simulink model "HIL_2"  (R2024a)
settings: Solver=ode3  StartTime=0.0  StopTime=inf  FixedStep=0.01  RelTol=1e-3  EnableMultiTasking=on
undefined symbols (not defined in the file or in its folder): k
libraries: arduinolib x3, simulink x2
settings Model: FPTRunName=Active  SimulationMode=external  ExtModeTrigDuration=2  Creator=refai  LastModifiedBy=refai
settings SolverCC: AlgebraicLoopSolver=TrustRegion  AutoInsertRateTranBlk=on
settings DataIOCC: LimitDataPoints=on  SaveFormat=Array
settings OptimizationCC: ReuseModelBlockBuffer=off  ExpressionDepthLimit=2147483647  LifeSpan=Inf  MaxStackSize=64
settings DebuggingCC: UnderspecifiedInitializationDetection=Classic  MergeDetectMultiDrivingBlocksExec=none  FcnCallInpInsideContextMsg=warning  UnconnectedInputMsg=warning  UnconnectedOutputMsg=warning  UnconnectedLineMsg=warning  AllowSymbolicDim=off  StateNameClashWarn=warning  SFUnexpectedBacktrackingDiag=warning  SFNoUnconditionalDefaultTransitionDiag=warning  SFExecutionAtInitializationDiag=none  ArithmeticOperatorsInVariantConditions=warning
settings HardwareCC: ProdBitPerInt=16  ProdBitPerPointer=16  ProdBitPerSizeT=16  ProdBitPerPtrDiffT=16  ProdLargestAtomicFloat=None  ProdWordSize=8  ProdHWDeviceType=Atmel->AVR
settings ModelReferenceCC: EnableRefExpFcnMdlSchedulingChecks=on  PropagateSignalLabelsOutOfModel=off
settings SFSimCC: SimUseLocalCustomCode=off  CustomCodeUndefinedFunction=UseInterfaceOnly
settings RTWCC: Description=Embedded Coder  SystemTargetFile=ert.tlc  HardwareBoard=Arduino Uno  TemplateMakefile=ert_default_tmf  GenerateReport=on  RTWVerbose=off  RTWUseLocalCustomCode=off  Toolchain=Arduino AVR  BuildConfiguration=Faster Runs  LaunchReport=on  GPUComputeCapability=3.5
settings CodeAppCC: ForceParamTrailComments=on  OperatorAnnotations=on  StateflowObjectComments=on  MATLABSourceComments=on
settings ERTTargetCC: MultiwordLength=2048  ERTCustomFileBanners=off  SupportContinuousTime=on  SupportNonInlinedSFcns=on  RemoveResetFunc=off  SupportVariableSizeSignals=on  ModelStepFunctionPrototypeControlCompliant=off  ExtMode=on  ExtModeTransport=3  ExtModeStaticAlloc=on  ExtModeAutomaticAllocSize=off  ExtModeStaticAllocSize=250  ExtModeMexFile=ext_xcp  ExtModeMexArgs=0 8 115200  ExtModeIntrfLevel=Level2 - Open
settings ConfigComp: CovMetricSettings=dw  CovSaveCumulativeToWorkspaceVar=on  CovSaveSingleToWorkspaceVar=on  CovExternalEMLEnable=off  CovSFcnEnable=off

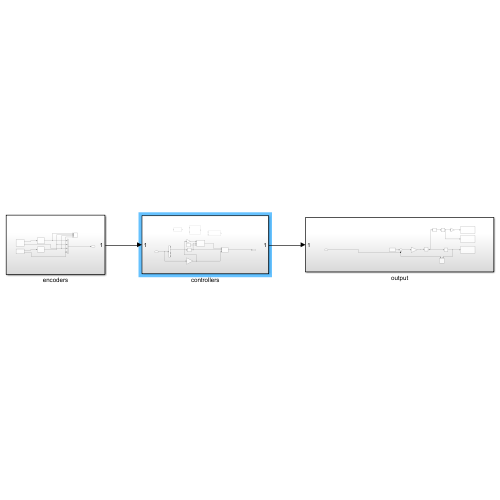
[thumbnail: Simulink's stored preview of the top-level diagram]
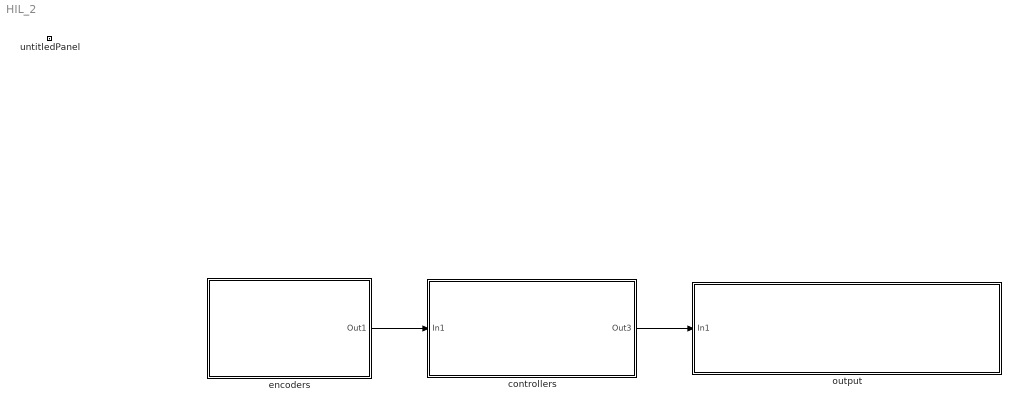
== system HIL_2 ==
  controllers : Subsystem
  encoders : Subsystem
  output : Subsystem
  untitledPanel : Subsystem  Tag=HiddenForWebPanel  IsWebBlockPanel=on
  wires:
  encoders/1(Out1) -> controllers/1(In1)
  controllers/1(Out3) -> output/1(In1)

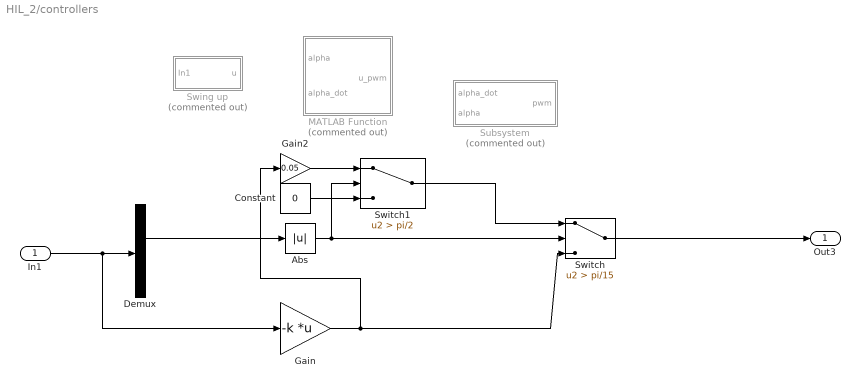
== system HIL_2/controllers ==
  In1 : Inport
  Abs : Abs  SaturateOnIntegerOverflow=off
  Constant : Constant  Value=0
  Demux : Demux
  Gain : Gain  Gain=-k  Multiplication=Matrix(K*u) (u vector)  ParamDataTypeStr=single  OutDataTypeStr=single
  Gain2 : Gain  Gain=0.05
  MATLAB Function : MATLAB Function  Commented=on  TreatAsAtomicUnit=on
  Subsystem : Subsystem  Commented=on
  Swing up : Subsystem  Commented=on
  Switch : Switch  Criteria=u2 > Threshold  Threshold=pi/15  SaturateOnIntegerOverflow=off  InputSameDT=off
  Switch1 : Switch  Criteria=u2 > Threshold  Threshold=pi/2  SaturateOnIntegerOverflow=off  InputSameDT=off
  Out3 : Outport
  wires:
  Gain/1 -> Gain2/1, Switch/3
  Abs/1 -> Switch1/2, Switch/2
  Demux/2 -> Abs/1
  In1/1 -> Demux/1, Gain/1
  Switch/1 -> Out3/1
  Gain2/1 -> Switch1/1
  Constant/1 -> Switch1/3
  Switch1/1 -> Switch/1

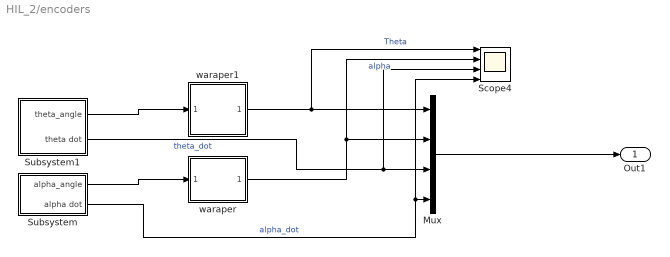
== system HIL_2/encoders ==
  Mux : Mux
  Scope4 : Scope  NumInputPorts=4
  Subsystem : Subsystem
  Subsystem1 : Subsystem
  waraper : Subsystem
  waraper1 : Subsystem
  Out1 : Outport
  wires:
  Subsystem1/2(theta dot) -> Scope4/3, Mux/3  "theta_dot"
  Subsystem/2(alpha dot) -> Mux/4, Scope4/4  "alpha_dot"
  waraper/1(Output) -> Mux/2, Scope4/2  "alpha"
  Subsystem1/1(theta_angle) -> waraper1/1(Input)
  waraper1/1(Output) -> Scope4/1, Mux/1  "Theta"
  Subsystem/1(alpha_angle) -> waraper/1(Input)
  Mux/1 -> Out1/1

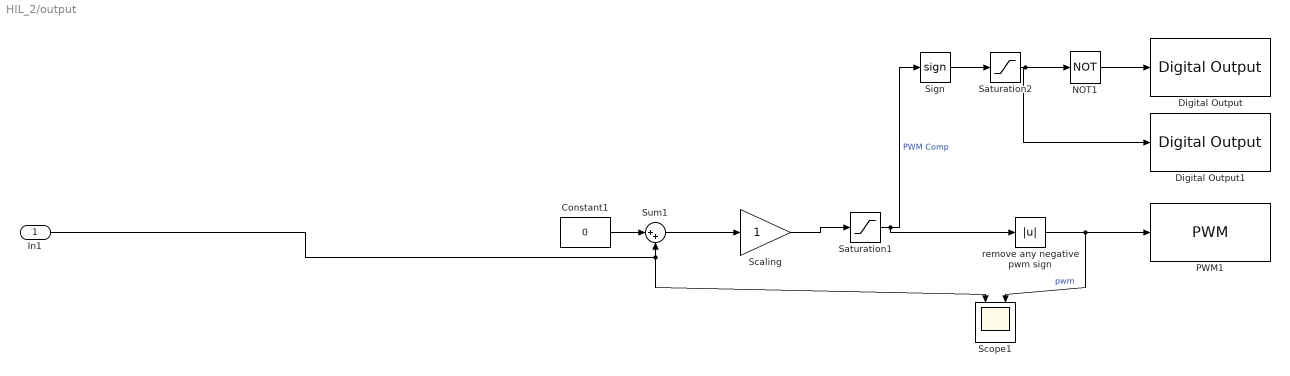
== system HIL_2/output ==
  In1 : Inport
  Constant1 : Constant  Value=0
  Digital Output : arduinolib/Digital Output  pinNumber=7  Direction=output  blockPlatform=arduino
  Digital Output1 : arduinolib/Digital Output  pinNumber=8  Direction=output  blockPlatform=arduino
  NOT1 : Logic  Operator=NOT  IconShape=distinctive  AllPortsSameDT=off  OutDataTypeStr=boolean
  PWM1 : arduinolib/PWM  pinNumber=9  frequencyType=Default  desiredFrequency=490.2  achievableFrequency=490.2
  Saturation1 : Saturate  UpperLimit=255  LowerLimit=-255
  Saturation2 : Saturate  UpperLimit=1  LowerLimit=0
  Scaling : Gain
  Scope1 : Scope  NumInputPorts=2
  Sign : Signum
  Sum1 : Sum  Inputs=|++
  remove any negative pwm sign : Abs  SaturateOnIntegerOverflow=off
  wires:
  Saturation2/1 -> Digital Output1/1, NOT1/1
  Scaling/1 -> Saturation1/1
  NOT1/1 -> Digital Output/1
  Sum1/1 -> Scaling/1
  Sign/1 -> Saturation2/1
  Saturation1/1 -> remove any negative pwm sign/1, Sign/1  "PWM Comp"
  In1/1 -> Scope1/1, Sum1/2
  remove any negative pwm sign/1 -> PWM1/1, Scope1/2  "pwm"
  Constant1/1 -> Sum1/1

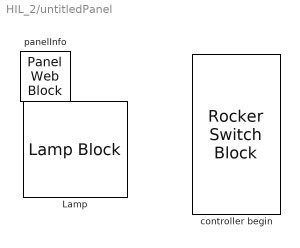
== system HIL_2/untitledPanel ==
  Lamp : LampBlock  Tag=HiddenForWebPanel  PanelInfo="{\"height\":158,\"left\":30,\"panelId\":\"panelId-8c924346-006a-4594-a17e-8cf792d8abfa\",\"top\":107,\"type\":\"panelChild\",\"version\":\"2019b\",\"width\":171,\"zIndex\":1500002}"  LabelPosition=Hide
  controller begin : RockerSwitchBlock  Tag=HiddenForWebPanel  PanelInfo="{\"height\":263,\"left\":308,\"panelId\":\"panelId-8c924346-006a-4594-a17e-8cf792d8abfa\",\"top\":30,\"type\":\"panelChild\",\"version\":\"2019b\",\"width\":145,\"zIndex\":1500004}"
      settings: Values={{'Off', 'On'}, [0 1]}
  panelInfo : PanelWebBlock  Tag=HiddenForWebPanel  PanelInfo="{\"compacted\":false,\"height\":329,\"isActiveTab\":true,\"left\":505,\"name\":\"Panel\",\"panelId\":\"panelId-8c924346-006a-4594-a17e-8cf792d8abfa\",\"popoutData\":{\"height\":0,\"left\":0,\"maximized\":false,\"top\":0,\"width\":0},\"popoutMode\":\"component\",\"tabIndex\":0,\"tabbedSetId\":\"tabbedSet4765928719\",\"top\":34,\"type\":\"panel\",\"version\":\"2019b\",\"visible\":true,\"width\":489,\"zIndex\":1500002}"  PanelSnapshot=<binary blob, 652 chars, not shown>

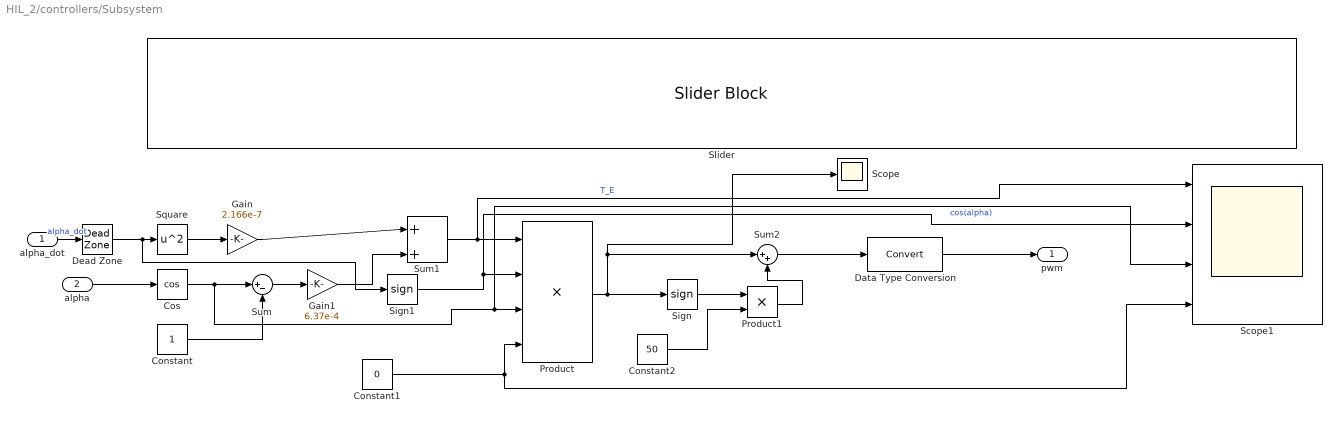
== system HIL_2/controllers/Subsystem ==
  alpha_dot : Inport
  alpha : Inport  Port=2
  Constant : Constant
  Constant1 : Constant  Value=0
  Constant2 : Constant  Value=50
  Cos : Trigonometry  Operator=cos
  Data Type Conversion : DataTypeConversion  SaturateOnIntegerOverflow=off  RndMeth=Floor
  Dead Zone : DeadZone
  Gain : Gain  Gain=2.166e-7
  Gain1 : Gain  Gain=6.37e-4
  Product : Product  Inputs=4
  Product1 : Product
  Scope : Scope
  Scope1 : Scope  NumInputPorts=4
  Sign : Signum
  Sign1 : Signum
  Slider : SliderBlock  ScaleMin=-100000  ScaleMax=100000
  Square : Math  Operator=square
  Sum : Sum  Inputs=|+-
  Sum1 : Sum  Inputs=|++
  Sum2 : Sum  Inputs=|++
  pwm : Outport  OutDataTypeStr=single
  wires:
  alpha_dot/1 -> Dead Zone/1  "alpha_dot"
  Square/1 -> Gain/1
  alpha/1 -> Cos/1
  Cos/1 -> Scope1/3, Product/3, Sum/1  "cos(alpha)"
  Constant/1 -> Sum/2
  Sum/1 -> Gain1/1
  Gain/1 -> Sum1/1
  Gain1/1 -> Sum1/2
  Sum1/1 -> Scope1/1, Product/1  "T_E"
  Constant1/1 -> Product/4, Scope1/4
  Product/1 -> Sign/1, Sum2/1, Scope/1
  Constant2/1 -> Product1/2
  Sign/1 -> Product1/1
  Product1/1 -> Sum2/2
  Sum2/1 -> Data Type Conversion/1
  Data Type Conversion/1 -> pwm/1
  Sign1/1 -> Scope1/2, Product/2
  Dead Zone/1 -> Sign1/1, Square/1

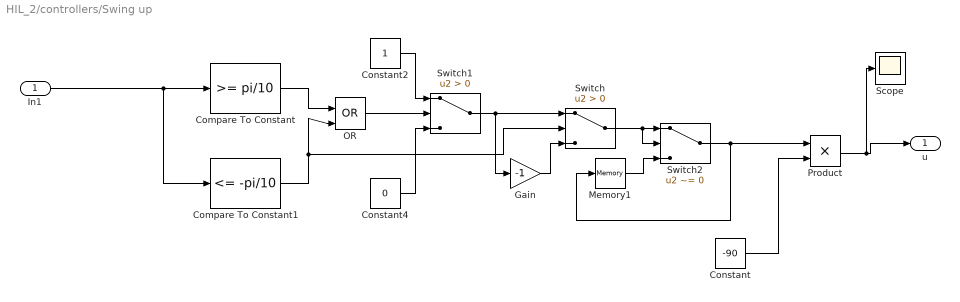
== system HIL_2/controllers/Swing up ==
  In1 : Inport
  Compare To Constant : simulink/Logic and Bit Operations/Compare To Constant  relop=>=  const=pi/10  OutDataTypeStr=boolean
  Compare To Constant1 : simulink/Logic and Bit Operations/Compare To Constant  relop=<=  const=-pi/10  OutDataTypeStr=boolean
  Constant : Constant  Value=-90
  Constant2 : Constant
  Constant4 : Constant  Value=0
  Gain : Gain  Gain=-1
  Memory1 : Memory  InitialCondition=1
  OR : Logic  Operator=OR  IconShape=distinctive  AllPortsSameDT=off  OutDataTypeStr=boolean
  Product : Product
  Scope : Scope
  Switch : Switch  Criteria=u2 > Threshold  SaturateOnIntegerOverflow=off  InputSameDT=off
  Switch1 : Switch  Criteria=u2 > Threshold  SaturateOnIntegerOverflow=off  InputSameDT=off
  Switch2 : Switch  Criteria=u2 ~= 0  SaturateOnIntegerOverflow=off  InputSameDT=off
  u : Outport
  wires:
  Switch1/1 -> Gain/1, Switch/1
  In1/1 -> Compare To Constant1/1, Compare To Constant/1
  Constant4/1 -> Switch1/3
  Constant2/1 -> Switch1/1
  Compare To Constant1/1 -> Switch/2, OR/2
  Compare To Constant/1 -> OR/1
  Gain/1 -> Switch/3
  OR/1 -> Switch1/2
  Constant/1 -> Product/2
  Switch/1 -> Switch2/2, Switch2/1
  Product/1 -> Scope/1, u/1
  Switch2/1 -> Product/1, Memory1/1
  Memory1/1 -> Switch2/3

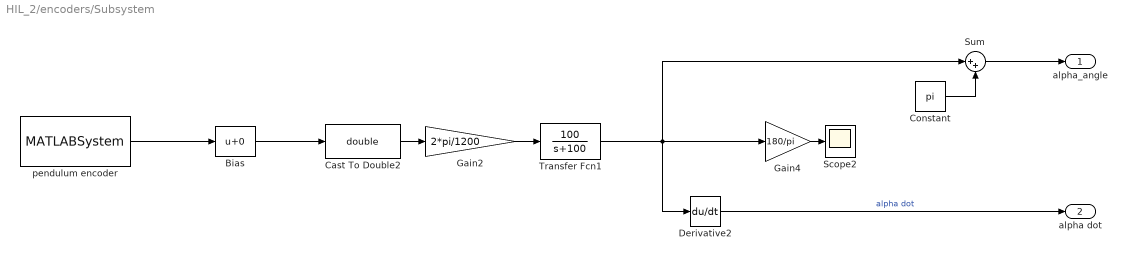
== system HIL_2/encoders/Subsystem ==
  Bias : Bias  SaturateOnIntegerOverflow=off
  Cast To Double2 : DataTypeConversion  OutDataTypeStr=double  SaturateOnIntegerOverflow=off  RndMeth=Floor
  Constant : Constant  Value=pi
  Derivative2 : Derivative
  Gain2 : Gain  Gain=2*pi/1200
  Gain4 : Gain  Gain=180/pi
  Scope2 : Scope
  Sum : Sum  Inputs=|++
  Transfer Fcn1 : TransferFcn  Numerator=[100]  Denominator=[1 100]
  pendulum encoder : MATLABSystem  System=Encoder_arduino  Encoder=0  PinA=3  PinB=5  SampleTime=0.01
      mask Type: Encoder_arduino
      mask Display:
      | disp('Encoder');
      | port_label('output',1,'y');
  alpha_angle : Outport
  alpha dot : Outport  Port=2
  wires:
  Transfer Fcn1/1 -> Sum/1, Gain4/1, Derivative2/1
  Gain2/1 -> Transfer Fcn1/1
  pendulum encoder/1 -> Bias/1
  Constant/1 -> Sum/2
  Gain4/1 -> Scope2/1
  Bias/1 -> Cast To Double2/1
  Cast To Double2/1 -> Gain2/1
  Sum/1 -> alpha_angle/1
  Derivative2/1 -> alpha dot/1  "alpha dot"

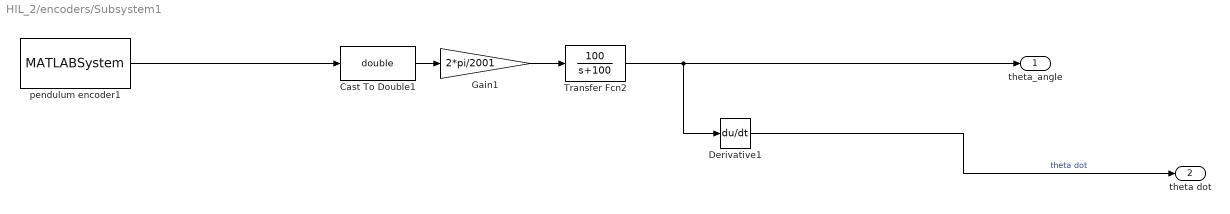
== system HIL_2/encoders/Subsystem1 ==
  Cast To Double1 : DataTypeConversion  OutDataTypeStr=double  SaturateOnIntegerOverflow=off  RndMeth=Floor
  Derivative1 : Derivative
  Gain1 : Gain  Gain=2*pi/2001
  Transfer Fcn2 : TransferFcn  Numerator=[100]  Denominator=[1 100]
  pendulum encoder1 : MATLABSystem  System=Encoder_arduino  Encoder=1  PinA=2  PinB=4  SampleTime=0.01
      mask Type: Encoder_arduino
      mask Display:
      | disp('Encoder');
      | port_label('output',1,'y');
  theta_angle : Outport
  theta dot : Outport  Port=2
  wires:
  Derivative1/1 -> theta dot/1  "theta dot"
  Transfer Fcn2/1 -> theta_angle/1, Derivative1/1
  pendulum encoder1/1 -> Cast To Double1/1
  Gain1/1 -> Transfer Fcn2/1
  Cast To Double1/1 -> Gain1/1

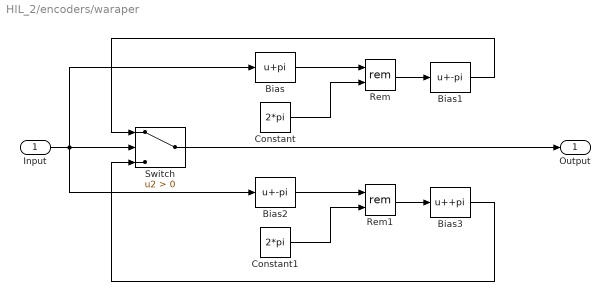
== system HIL_2/encoders/waraper ==
  Input : Inport
  Bias : Bias  Bias=pi  SaturateOnIntegerOverflow=off
  Bias1 : Bias  Bias=-pi  SaturateOnIntegerOverflow=off
  Bias2 : Bias  Bias=-pi  SaturateOnIntegerOverflow=off
  Bias3 : Bias  Bias=+pi  SaturateOnIntegerOverflow=off
  Constant : Constant  Value=2*pi
  Constant1 : Constant  Value=2*pi
  Rem : Math  Operator=rem
  Rem1 : Math  Operator=rem
  Switch : Switch  Criteria=u2 > Threshold  SaturateOnIntegerOverflow=off  InputSameDT=off
  Output : Outport
  wires:
  Constant/1 -> Rem/2
  Bias/1 -> Rem/1
  Input/1 -> Bias/1, Bias2/1, Switch/2
  Bias3/1 -> Switch/3
  Bias2/1 -> Rem1/1
  Rem1/1 -> Bias3/1
  Constant1/1 -> Rem1/2
  Switch/1 -> Output/1
  Rem/1 -> Bias1/1
  Bias1/1 -> Switch/1

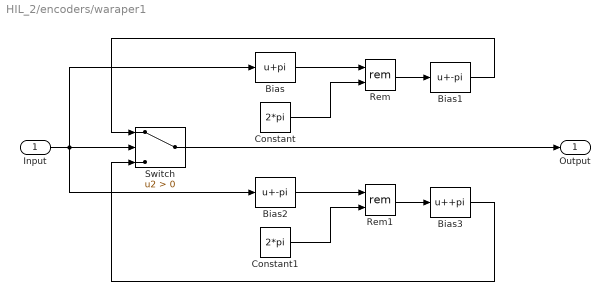
== system HIL_2/encoders/waraper1 ==
  Input : Inport
  Bias : Bias  Bias=pi  SaturateOnIntegerOverflow=off
  Bias1 : Bias  Bias=-pi  SaturateOnIntegerOverflow=off
  Bias2 : Bias  Bias=-pi  SaturateOnIntegerOverflow=off
  Bias3 : Bias  Bias=+pi  SaturateOnIntegerOverflow=off
  Constant : Constant  Value=2*pi
  Constant1 : Constant  Value=2*pi
  Rem : Math  Operator=rem
  Rem1 : Math  Operator=rem
  Switch : Switch  Criteria=u2 > Threshold  SaturateOnIntegerOverflow=off  InputSameDT=off
  Output : Outport
  wires:
  Constant/1 -> Rem/2
  Bias/1 -> Rem/1
  Input/1 -> Bias/1, Bias2/1, Switch/2
  Bias3/1 -> Switch/3
  Bias2/1 -> Rem1/1
  Rem1/1 -> Bias3/1
  Constant1/1 -> Rem1/2
  Switch/1 -> Output/1
  Rem/1 -> Bias1/1
  Bias1/1 -> Switch/1

== matlab function HIL_2/controllers/MATLAB Function ==
  data: alpha input; u_pwm output; alpha_dot input
function u_pwm = aggressive_swingup(alpha, alpha_dot)
    % --- INITIALIZATION ---
    % We use 'single' to ensure compatibility with Arduino hardware
    u_pwm = single(0);
    
    % --- CONFIGURATION ---
    % Power gain: 200-255 is aggressive for a 13g pendulum
    % If the motor 'brakes' instead of 'pushes', change this to -220
    ke = single(220); 
    
    % --- RANGE LOGIC (QUADRANT CONTROL) ---
    % Since alpha is wrapped between -pi and pi, the bottom half is 
    % split into two ranges
    
    % Range 1: Bottom-Right (90 to 180 degrees)
    range_right = (alpha > 1.57) && (alpha <= 3.1416);
    
    % Range 2: Bottom-Left (-180 to -90 degrees)
    range_left = (alpha >= -3.1416) && (alpha < -1.57);
    
    % --- EXECUTION ---
    % Check if the pendulum is in the 'Push Zone' (bottom half)
    if (range_right || range_left)
        
        % Filter out the fake velocity spike caused by the pi to -pi jump
        % If velocity is too high (>100 rad/s), it is a sensor glitch
        is_real_motion = (abs(alpha_dot) > 0.5) && (abs(alpha_dot) < 100);
        
        if is_real_motion
            % Aggressive 'Punch': Move theta in the direction of alpha_dot
            u_pwm = single(sign(alpha_dot) * ke);
        end
        
    end
    
    % --- FINAL SAFETY SATURATION ---
    % Limits signal to valid Arduino PWM range [-255, 255]
    if u_pwm > 255
        u_pwm = single(255);
    elseif u_pwm < -255
        u_pwm = single(-255);
    end
end
